simulink model "MPC_Simulink"  (R2023b)
settings: Solver=FixedStepAuto  StartTime=0.0  StopTime=inf  RelTol=1e-3
libraries: arduinolib x2, mpclib x1
settings Model: ExtModeTrigDuration=2  Creator=vagge  LastModifiedBy=vagge
settings OptimizationCC: EnhancedBackFolding=on  PassReuseOutputArgsAs=Individual arguments  ZeroExternalMemoryAtStartup=off  ZeroInternalMemoryAtStartup=off  MaxStackSize=64  OptimizeBlockOrder=speed  DifferentSizesBufferReuse=on  OptimizationCustomize=off  EfficientTunableParamExpr=on
settings DebuggingCC: ParameterOverflowMsg=none  ParameterPrecisionLossMsg=none  ParameterTunabilityLossMsg=error
settings HardwareCC: ProdBitPerInt=16  ProdBitPerPointer=16  ProdBitPerSizeT=16  ProdBitPerPtrDiffT=16  ProdLargestAtomicFloat=None  ProdWordSize=8  ProdHWDeviceType=Atmel->AVR  UseEmbeddedCoderFeatures=off  UseSimulinkCoderFeatures=off
settings SFSimCC: MATLABDynamicMemAlloc=off
settings RTWCC: Description=Embedded Coder  SystemTargetFile=ert.tlc  HardwareBoard=Arduino Uno  TemplateMakefile=ert_default_tmf  Toolchain=Arduino AVR
settings CodeAppCC: ForceParamTrailComments=on  IgnoreCustomStorageClasses=off  OperatorAnnotations=on  SimulinkDataObjDesc=on  SFDataObjDesc=on  InsertBlockDesc=on
settings ERTTargetCC: SupportContinuousTime=on  SupportNonInlinedSFcns=on  SupportVariableSizeSignals=on  ExtModeTransport=3  ExtModeStaticAlloc=on  ExtModeAutomaticAllocSize=off  ExtModeStaticAllocSize=250  ExtModeMexFile=ext_xcp  ExtModeIntrfLevel=Level2 - Open

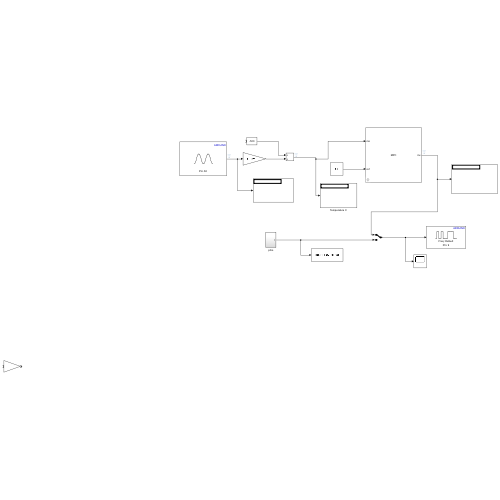
[thumbnail: Simulink's stored preview of the top-level diagram]
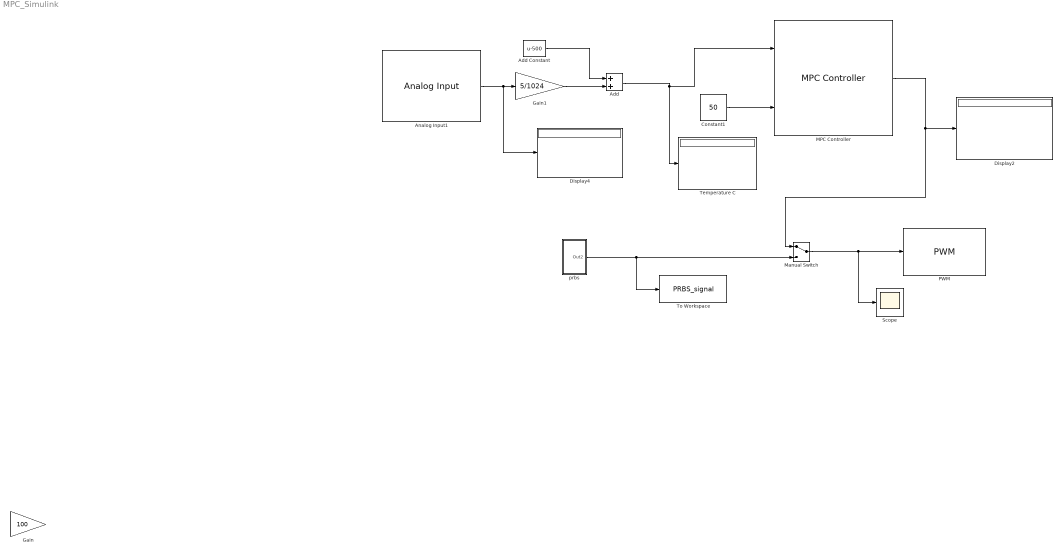
== system MPC_Simulink ==
  Add : Sum
  Add Constant : Bias  Bias=-500  SaturateOnIntegerOverflow=off
  Analog Input1 : arduinolib/Analog Input  pinNumber=5  ReadResultsOnly=off  ConversionTriggerSource=Software  ExternalTriggerType=uint32( 0 )  OutputDataType=uint16  EnableConversionCompleteNotify=off  EnableOuputStatus=off  SampleTime=-1  blockPlatform=arduino
  Constant1 : Constant  Value=50
  Display2 : Display
  Display4 : Display
  Gain : Gain  Gain=100
  Gain1 : Gain  Gain=5/1024
  MPC Controller : mpclib/MPC Controller  SCDEnableBlockLinearizationSpecification=on  mpcobj=mpc1  is_multiple=0  enable_value=0  return_u0=off  updateMPCinCallerWorkspace=on  md_inport=off  mv_inport=off  uref_inport=off  return_cost=off  return_mvseq=off  return_qpstatus=off  return_xseq=off  return_state=off  return_ovseq=off  state_inport=off  umin_inport=off  umax_inport=off  ymin_inport=off  ymax_inport=off  cc_inport=off  ywt_inport=off  uwt_inport=off  duwt_inport=off  rhoeps_inport=off  pm_inport=off  MaximumP=10  HorizonChoice=FixedHorizon  n_ts=100  n_p=10  n_mv=1  n_md=0  n_ud=0  n_mo=1  n_uo=0  BlockDataType=double  SampleTimeInherited=off  switch_inport=off
  Manual Switch : ManualSwitch
  PWM : arduinolib/PWM  pinNumber=9  frequencyType=Default  desiredFrequency=490.2  achievableFrequency=490.2
  Scope : Scope
  Temperature C : Display
  To Workspace : ToWorkspace  VariableName=PRBS_signal  SaveFormat=Timeseries  SampleTime=-1
  prbs : Subsystem
  wires:
  Constant1/1 -> MPC Controller/2
  MPC Controller/1 -> Manual Switch/1, Display2/1
  prbs/1(Out2) -> Manual Switch/2, To Workspace/1
  Manual Switch/1 -> Scope/1, PWM/1
  Gain1/1 -> Add/2
  Analog Input1/1 -> Display4/1, Gain1/1
  Add/1 -> MPC Controller/1, Temperature C/1
  Add Constant/1 -> Add/1

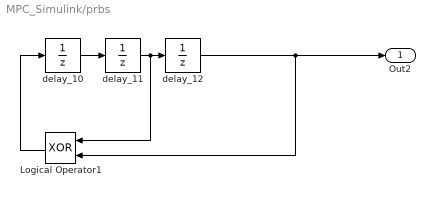
== system MPC_Simulink/prbs ==
  Logical Operator1 : Logic  Operator=XOR  AllPortsSameDT=off  OutDataTypeStr=boolean
  delay_10 : UnitDelay  InitialCondition=1
  delay_11 : UnitDelay  InitialCondition=1  SampleTime=-1
  delay_12 : UnitDelay  InitialCondition=1  SampleTime=-1
  Out2 : Outport
  wires:
  delay_11/1 -> delay_12/1, Logical Operator1/1
  delay_12/1 -> Logical Operator1/2, Out2/1
  delay_10/1 -> delay_11/1
  Logical Operator1/1 -> delay_10/1
